simulink model "expe2_model_v1"  (R2019b)
settings: Solver=VariableStepAuto  StartTime=0.0  StopTime=time  RelTol=1e-3
values from neighbouring files (symbols this model uses):
  Gs = tf(1, [1 3 3 1 0])    [expe1_params_v1.m]    (also in expe1_params_v2.m; expe2_params.m = tf([-1 0.4], [1 0.5 0.04]))
  half_time = time/2    (= 25)    [expe1_params_v1.m]    (also in expe1_params_v2.m = 250; expe2_params.m = 50)
  system1 = ModelPID(a1, a2, b0, b1, damp_coeff1, wn1, lambda)    [expe2_params.m]
  system2 = ModelPID(a1, a2, b0, b1, damp_coeff2, wn2, lambda)    [expe2_params.m]
  system3 = ModelPID(a1, a2, b0, b1, damp_coeff3, wn3, lambda)    [expe2_params.m]
settings Model: Creator=adityaaaap  LastModifiedBy=adityaaaap

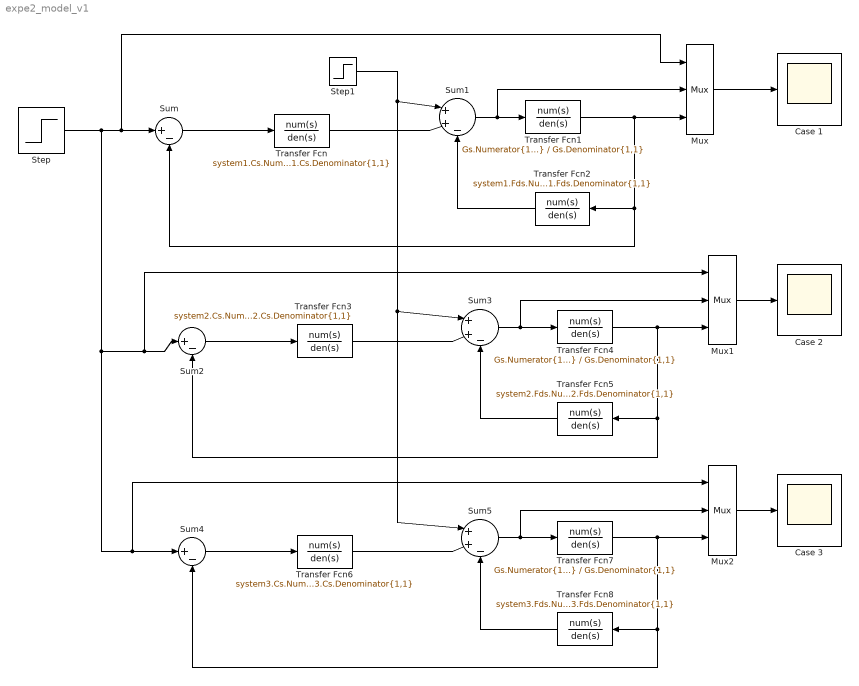
== system expe2_model_v1 ==
  Case 1 : Scope
  Case 2 : Scope
  Case 3 : Scope
  Mux : Mux  Inputs=3
  Mux1 : Mux  Inputs=3
  Mux2 : Mux  Inputs=3
  Step : Step  Time=0  After=3  SampleTime=0.1
  Step1 : Step  Time=half_time  SampleTime=0
  Sum : Sum  Inputs=|+-
  Sum1 : Sum  Inputs=|++-
  Sum2 : Sum  Inputs=|+-
  Sum3 : Sum  Inputs=|++-
  Sum4 : Sum  Inputs=|+-
  Sum5 : Sum  Inputs=|++-
  Transfer Fcn : TransferFcn  Numerator=system1.Cs.Numerator{1,1}  Denominator=system1.Cs.Denominator{1,1}
  Transfer Fcn1 : TransferFcn  Numerator=Gs.Numerator{1,1}  Denominator=Gs.Denominator{1,1}
  Transfer Fcn2 : TransferFcn  Numerator=system1.Fds.Numerator{1,1}  Denominator=system1.Fds.Denominator{1,1}
  Transfer Fcn3 : TransferFcn  Numerator=system2.Cs.Numerator{1,1}  Denominator=system2.Cs.Denominator{1,1}
  Transfer Fcn4 : TransferFcn  Numerator=Gs.Numerator{1,1}  Denominator=Gs.Denominator{1,1}
  Transfer Fcn5 : TransferFcn  Numerator=system2.Fds.Numerator{1,1}  Denominator=system2.Fds.Denominator{1,1}
  Transfer Fcn6 : TransferFcn  Numerator=system3.Cs.Numerator{1,1}  Denominator=system3.Cs.Denominator{1,1}
  Transfer Fcn7 : TransferFcn  Numerator=Gs.Numerator{1,1}  Denominator=Gs.Denominator{1,1}
  Transfer Fcn8 : TransferFcn  Numerator=system3.Fds.Numerator{1,1}  Denominator=system3.Fds.Denominator{1,1}
  wires:
  Sum/1 -> Transfer Fcn/1
  Transfer Fcn/1 -> Sum1/2
  Sum1/1 -> Mux/2, Transfer Fcn1/1
  Transfer Fcn1/1 -> Sum/2, Transfer Fcn2/1, Mux/3
  Transfer Fcn2/1 -> Sum1/3
  Mux/1 -> Case 1/1
  Transfer Fcn3/1 -> Sum3/2
  Transfer Fcn5/1 -> Sum3/3
  Mux1/1 -> Case 2/1
  Sum3/1 -> Mux1/2, Transfer Fcn4/1
  Sum2/1 -> Transfer Fcn3/1
  Transfer Fcn4/1 -> Sum2/2, Transfer Fcn5/1, Mux1/3
  Step/1 -> Mux2/1, Sum4/1, Mux1/1, Sum2/1, Mux/1, Sum/1
  Mux2/1 -> Case 3/1
  Transfer Fcn6/1 -> Sum5/2
  Sum5/1 -> Mux2/2, Transfer Fcn7/1
  Transfer Fcn8/1 -> Sum5/3
  Step1/1 -> Sum5/1, Sum3/1, Sum1/1
  Transfer Fcn7/1 -> Sum4/2, Transfer Fcn8/1, Mux2/3
  Sum4/1 -> Transfer Fcn6/1
